simulink model "start_mdl_dc_motor2"  (R2013b)
settings: Solver=ode3  StartTime=0.0  StopTime=1  FixedStep=1e-3  RelTol=1e-3
values from neighbouring files (symbols this model uses):
  b = a(n+1)    [Batherwort_polinom_coefficients.m]    (also in Modal_control.m; Niewton_coeff.m; lab7_script.m)
  ce = (Un - In*R)/wn    (= 0.301701587302)    [params.m]    (also in params_fun.m)
  cm = Mn/In    (= 0.212068965517)    [params.m]    (also in params_fun.m)
  Jm = 0.59*10^(-4)    (= 5.9e-05)    [params.m]    (also in params_fun.m)
  K = place(A,B,p)    [Modal_control.m]    (also in lab7_script.m)
  L = 130*10^(-3)    (= 0.13)    [params.m]    (also in params_fun.m)
  R = 25.8    [params.m]    (also in params_fun.m)
settings Model: BufferReuse=off  Creator=user  LastModifiedBy=user
settings DataIOCC: LimitDataPoints=off
settings OptimizationCC: InlineParams=on  BufferReuse=off
settings DebuggingCC: InitInArrayFormatMsg=none

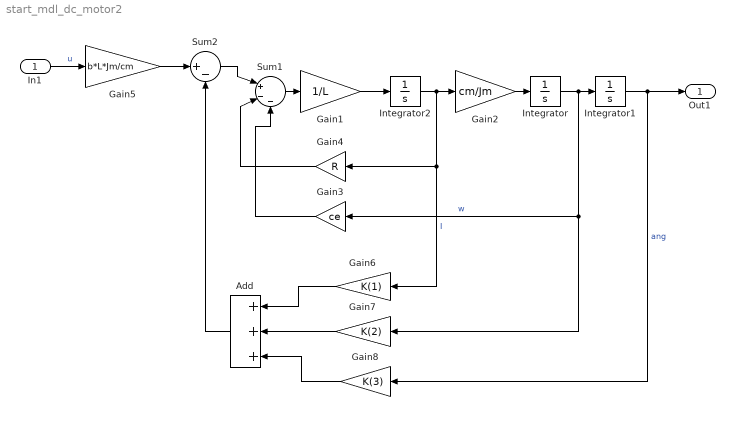
== system start_mdl_dc_motor2 ==
  In1 : Inport
  Add : Sum  Inputs=+++
  Gain1 : Gain  Gain=1/L
  Gain2 : Gain  Gain=cm/Jm
  Gain3 : Gain  Gain=ce
  Gain4 : Gain  Gain=R
  Gain5 : Gain  Gain=b*L*Jm/cm
  Gain6 : Gain  Gain=K(1)
  Gain7 : Gain  Gain=K(2)
  Gain8 : Gain  Gain=K(3)
  Integrator : Integrator
  Integrator1 : Integrator
  Integrator2 : Integrator
  Sum1 : Sum  Inputs=|+--
  Sum2 : Sum  Inputs=|+-
  Out1 : Outport
  wires:
  Integrator2/1 -> Gain6/1, Gain4/1, Gain2/1  "I"
  Gain2/1 -> Integrator/1
  Integrator/1 -> Gain7/1, Gain3/1, Integrator1/1  "w"
  Sum1/1 -> Gain1/1
  Integrator1/1 -> Out1/1, Gain8/1  "ang"
  Gain1/1 -> Integrator2/1
  Gain4/1 -> Sum1/2
  Gain3/1 -> Sum1/3
  Gain6/1 -> Add/1
  Gain7/1 -> Add/2
  Gain8/1 -> Add/3
  Add/1 -> Sum2/2
  Sum2/1 -> Sum1/1
  Gain5/1 -> Sum2/1
  In1/1 -> Gain5/1  "u"
